simulink model "vs2"  (R2021a)
settings: Solver=VariableStepAuto  StartTime=0.0  StopTime=inf  RelTol=1e-3
undefined symbols (not defined in the file): LF
libraries: instrumentseriallib x2
settings Model: Creator=Sergio  LastModifiedBy=Ravenelco

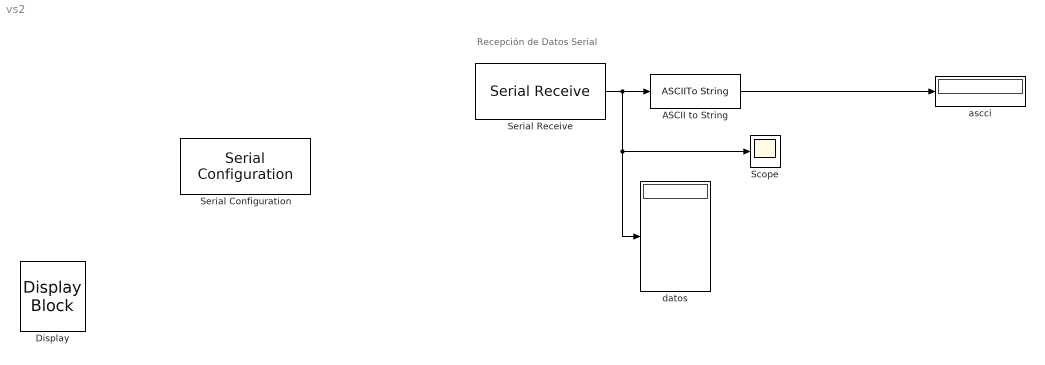
== system vs2 ==
  note: Recepción de Datos Serial
  ASCII to String : ASCIIToString
  Display : DisplayBlock  LabelPosition=Hide  Format=short  Transparency=1  Layout=Fill available space
  Scope : Scope
  "Serial Configuration " : instrumentseriallib/Serial Configuration  Priority=-200000  Port=COM12  ComPort=COM12  BaudRate=9600  DataBits=8  Parity=none  StopBits=1  ByteOrder=little-endian  FlowControl=none  Timeout=0.01  SimulateUsing=Interpreted execution  BlockInModel=on
  "Serial Receive " : instrumentseriallib/Serial Receive  Priority=1  Port=COM12  ComPort=COM12  DataType=uint8  SaveDataType=uint8  ToggleHeader=off  Header='V'  ToggleTerminator=off  Terminator=LF ('\n')  CustomTerminator=[]  ToggleDataSize=on  DataSize=[1]  EnableBlockingMode=on  ActionDataUnavailable=Output last received value  ActionWhenDataUnavailable=Output last received value  CustomValue=0  SampleTime=0.001  SimulateUsing=Interpreted execution  BlockInModel=on
  ascci : Display
  datos : Display
  wires:
  "Serial Receive "/1 -> Scope/1, datos/1, ASCII to String/1
  ASCII to String/1 -> ascci/1
